simulink model "first_a"  (R2017a)
settings: Solver=VariableStepAuto  StartTime=0.0  StopTime=0.02  RelTol=1e-3
settings Model: Creator=user  LastModifiedBy=user

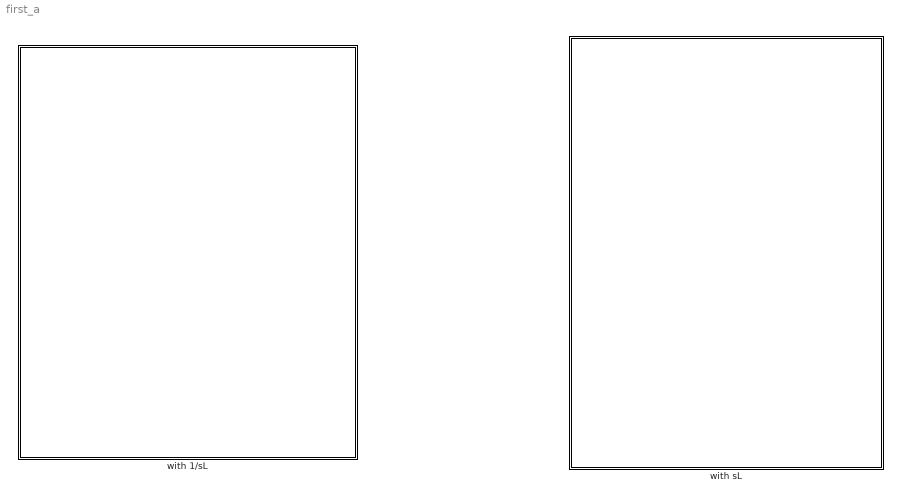
== system first_a ==
  with 1/sL : Subsystem
  with sL : Subsystem

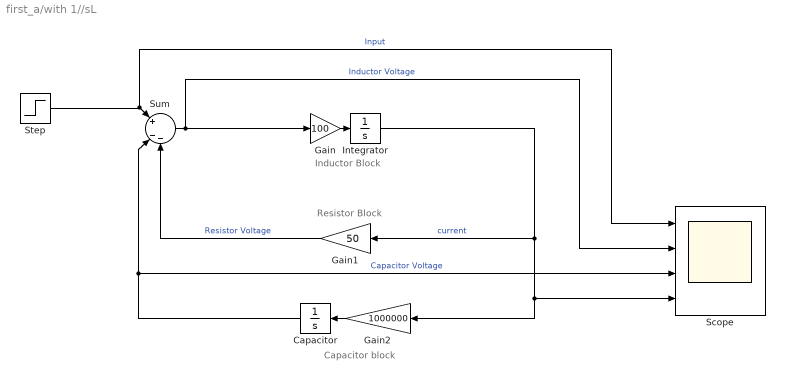
== system first_a/with 1//sL ==
  note: Capacitor block
  note: Resistor Block
  note: Inductor Block
  Capacitor : Integrator
  Gain : Gain  Gain=100
  Gain1 : Gain  Gain=50
  Gain2 : Gain  Gain=1000000
  Integrator : Integrator
  Scope : Scope  NumInputPorts=4
  Step : Step  Time=0.01  SampleTime=0
  Sum : Sum  Inputs=|+|--
  wires:
  Gain1/1 -> Sum/3  "Resistor Voltage"
  Integrator/1 -> Scope/4, Gain2/1, Gain1/1  "current"
  Step/1 -> Scope/1, Sum/1  "Input"
  Capacitor/1 -> Scope/3, Sum/2  "Capacitor Voltage"
  Sum/1 -> Scope/2, Gain/1  "Inductor Voltage"
  Gain2/1 -> Capacitor/1
  Gain/1 -> Integrator/1

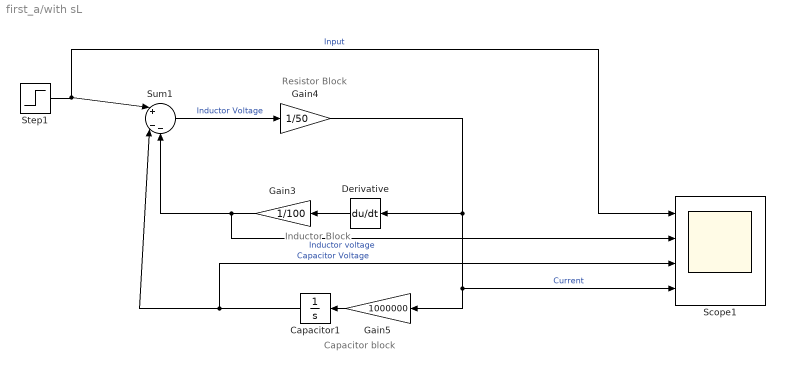
== system first_a/with sL ==
  note: Capacitor block
  note: Resistor Block
  note: Inductor Block
  Capacitor1 : Integrator
  Derivative : Derivative  CoefficientInTFapproximation=0
  Gain3 : Gain  Gain=1/100
  Gain4 : Gain  Gain=1/50
  Gain5 : Gain  Gain=1000000
  Scope1 : Scope  NumInputPorts=4
  Step1 : Step  Time=0  SampleTime=0
  Sum1 : Sum  Inputs=|+|--
  wires:
  Step1/1 -> Scope1/1, Sum1/1  "Input"
  Sum1/1 -> Gain4/1  "Inductor Voltage"
  Gain5/1 -> Capacitor1/1
  Derivative/1 -> Gain3/1
  Gain4/1 -> Gain5/1, Scope1/4, Derivative/1  "Current"
  Gain3/1 -> Scope1/2, Sum1/3  "Inductor voltage"
  Capacitor1/1 -> Scope1/3, Sum1/2  "Capacitor Voltage"
